simulink model "IEEE9Buses"  (R2024b)
settings: Solver=FixedStepAuto  StartTime=0  StopTime=5  FixedStep=1e-6  RelTol=1e-3
values from neighbouring files (symbols this model uses):
  SG_D_1_D = 0.01056    [SG9_parameters.m]
  SG_D_1_EnableSaturation = 0    [SG9_parameters.m]
  SG_D_1_f0 = 60    [SG9_parameters.m]
  SG_D_1_H = 7.5    [SG9_parameters.m]
  SG_D_1_K_A = 20    [SG9_parameters.m]
  SG_D_1_K_E = 1.000000e+1    (= 10)    [SG9_parameters.m]
  SG_D_1_K_F = 2.363    [SG9_parameters.m]
  SG_D_1_K_s = 5    [SG9_parameters.m]
  SG_D_1_R_a = 0.001088    [SG9_parameters.m]
  SG_D_1_S_A = 1    [SG9_parameters.m]
  SG_D_1_S_B = 0.103    [SG9_parameters.m]
  SG_D_1_S_N = 10.659857    [SG9_parameters.m]
  SG_D_1_SpeedPara = 200    [SG9_parameters.m]
  SG_D_1_T_0 = 0.720173    [SG9_parameters.m]
  SG_D_1_T_1 = 0.3    [SG9_parameters.m]
  SG_D_1_T_2 = 0.05    [SG9_parameters.m]
  SG_D_1_T_3 = 0.02    [SG9_parameters.m]
  SG_D_1_T_4 = 0.005    [SG9_parameters.m]
  SG_D_1_T_A = 0.02    [SG9_parameters.m]
  SG_D_1_T_dd = 8.000000e+0    (= 8)    [SG9_parameters.m]
  SG_D_1_T_ddd = 0.04    [SG9_parameters.m]
  SG_D_1_T_E = 0.314    [SG9_parameters.m]
  SG_D_1_T_F = 0.35    [SG9_parameters.m]
  SG_D_1_T_qd = 0.8    [SG9_parameters.m]
  SG_D_1_T_qdd = 0.02    [SG9_parameters.m]
  SG_D_1_T_speed = 0.1    [SG9_parameters.m]
  SG_D_1_T_w = 0.5    [SG9_parameters.m]
  SG_D_1_V_ref = 1.990276    [SG9_parameters.m]
  SG_D_1_w_ref = 376.991118    [SG9_parameters.m]
  SG_D_1_x_d = 1.9    [SG9_parameters.m]
  SG_D_1_x_dd = 0.302    [SG9_parameters.m]
  SG_D_1_x_ddd = 0.204    [SG9_parameters.m]
  SG_D_1_x_l = 0.05    [SG9_parameters.m]
  SG_D_1_x_q = 1.3    [SG9_parameters.m]
  SG_D_1_x_qd = 0.5    [SG9_parameters.m]
  SG_D_1_x_qdd = 0.3    [SG9_parameters.m]
  SG_D_2_D = 0.01056    [SG9_parameters.m]
  SG_D_2_EnableSaturation = 0    [SG9_parameters.m]
  SG_D_2_f0 = 60    [SG9_parameters.m]
  SG_D_2_H = 7.5    [SG9_parameters.m]
  SG_D_2_K_A = 20    [SG9_parameters.m]
  SG_D_2_K_E = 1.000000e+1    (= 10)    [SG9_parameters.m]
  SG_D_2_K_F = 2.363    [SG9_parameters.m]
  SG_D_2_K_s = 0.5    [SG9_parameters.m]
  SG_D_2_R_a = 0.001088    [SG9_parameters.m]
  SG_D_2_S_A = 1    [SG9_parameters.m]
  SG_D_2_S_B = 0.103    [SG9_parameters.m]
  SG_D_2_S_N = 10.659857    [SG9_parameters.m]
  SG_D_2_SpeedPara = 200    [SG9_parameters.m]
  SG_D_2_T_0 = 1.632913    [SG9_parameters.m]
  SG_D_2_T_1 = 0.2    [SG9_parameters.m]
  SG_D_2_T_2 = 0.05    [SG9_parameters.m]
  SG_D_2_T_3 = 0.02    [SG9_parameters.m]
  SG_D_2_T_4 = 0.005    [SG9_parameters.m]
  SG_D_2_T_A = 0.02    [SG9_parameters.m]
  SG_D_2_T_dd = 8.000000e+0    (= 8)    [SG9_parameters.m]
  SG_D_2_T_ddd = 0.04    [SG9_parameters.m]
  SG_D_2_T_E = 0.314    [SG9_parameters.m]
  SG_D_2_T_F = 0.35    [SG9_parameters.m]
  SG_D_2_T_qd = 0.8    [SG9_parameters.m]
  SG_D_2_T_qdd = 0.02    [SG9_parameters.m]
  SG_D_2_T_speed = 0.1    [SG9_parameters.m]
  SG_D_2_T_w = 0.5    [SG9_parameters.m]
  SG_D_2_V_ref = 2.662631    [SG9_parameters.m]
  SG_D_2_w_ref = 376.991118    [SG9_parameters.m]
  SG_D_2_x_d = 1.9    [SG9_parameters.m]
  SG_D_2_x_dd = 0.302    [SG9_parameters.m]
  SG_D_2_x_ddd = 0.204    [SG9_parameters.m]
  SG_D_2_x_l = 0.05    [SG9_parameters.m]
  SG_D_2_x_q = 1.3    [SG9_parameters.m]
  SG_D_2_x_qd = 0.5    [SG9_parameters.m]
  SG_D_2_x_qdd = 0.3    [SG9_parameters.m]
  SG_D_3_D = 0.01056    [SG9_parameters.m]
  SG_D_3_EnableSaturation = 0    [SG9_parameters.m]
  SG_D_3_f0 = 60    [SG9_parameters.m]
  SG_D_3_H = 7.5    [SG9_parameters.m]
  SG_D_3_K_A = 20    [SG9_parameters.m]
  SG_D_3_K_E = 1.000000e+1    (= 10)    [SG9_parameters.m]
  SG_D_3_K_F = 2.363    [SG9_parameters.m]
  SG_D_3_K_s = 0.5    [SG9_parameters.m]
  SG_D_3_R_a = 0.001088    [SG9_parameters.m]
  SG_D_3_S_A = 1    [SG9_parameters.m]
  SG_D_3_S_B = 0.103    [SG9_parameters.m]
  SG_D_3_S_N = 10.659857    [SG9_parameters.m]
  SG_D_3_SpeedPara = 200    [SG9_parameters.m]
  SG_D_3_T_0 = 0.850788    [SG9_parameters.m]
  SG_D_3_T_1 = 0.2    [SG9_parameters.m]
  SG_D_3_T_2 = 0.05    [SG9_parameters.m]
  SG_D_3_T_3 = 0.02    [SG9_parameters.m]
  SG_D_3_T_4 = 0.005    [SG9_parameters.m]
  SG_D_3_T_A = 0.02    [SG9_parameters.m]
  SG_D_3_T_dd = 8.000000e+0    (= 8)    [SG9_parameters.m]
  SG_D_3_T_ddd = 0.04    [SG9_parameters.m]
  SG_D_3_T_E = 0.314    [SG9_parameters.m]
  SG_D_3_T_F = 0.35    [SG9_parameters.m]
  SG_D_3_T_qd = 0.8    [SG9_parameters.m]
  SG_D_3_T_qdd = 0.02    [SG9_parameters.m]
  SG_D_3_T_speed = 0.1    [SG9_parameters.m]
  SG_D_3_T_w = 0.5    [SG9_parameters.m]
  SG_D_3_V_ref = 1.915682    [SG9_parameters.m]
  SG_D_3_w_ref = 376.991118    [SG9_parameters.m]
  SG_D_3_x_d = 1.9    [SG9_parameters.m]
  SG_D_3_x_dd = 0.302    [SG9_parameters.m]
  SG_D_3_x_ddd = 0.204    [SG9_parameters.m]
  SG_D_3_x_l = 0.05    [SG9_parameters.m]
  SG_D_3_x_q = 1.3    [SG9_parameters.m]
  SG_D_3_x_qd = 0.5    [SG9_parameters.m]
  SG_D_3_x_qdd = 0.3    [SG9_parameters.m]
(part 6 of 9)

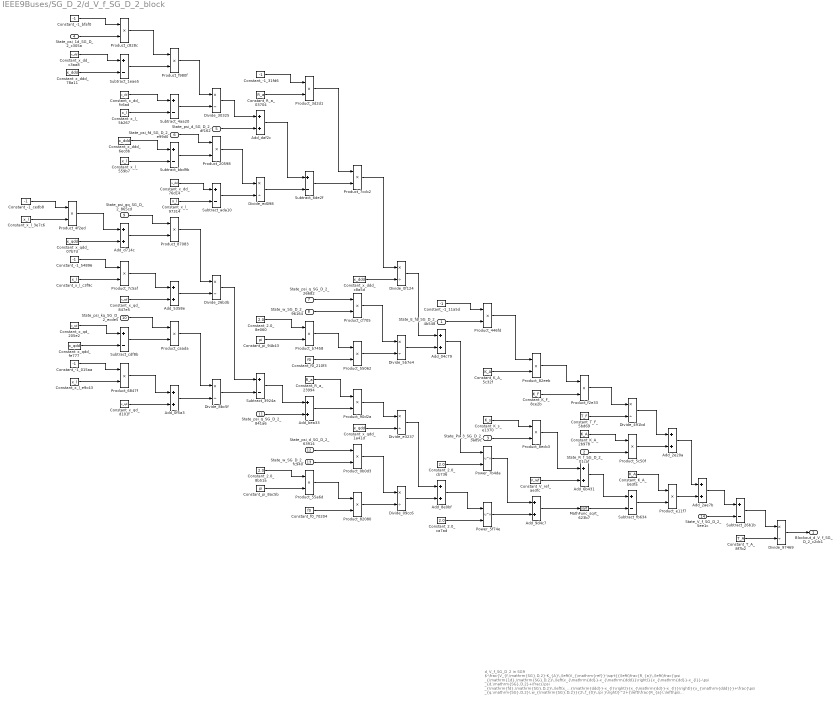
== system IEEE9Buses/SG_D_2/d_V_f_SG_D_2_block ==
  note: d_V_f_SG_D_2 in SG9
      | $-\frac{V_{f,\mathrm{SG},D,2}-K_{A}\,\left(V_{\mathrm{ref}}-\sqrt{{\left(\frac{R_{a}\,\left(\frac{\psi _{\mathrm{1d},\mathrm{SG},D,2}\,\left(x_{\mathrm{dd}}-x_{\mathrm{ddd}}\right)}{x_{\mathrm{dd}}-x_{l}}-\psi _{d,\mathrm{SG},D,2}+\frac{\psi _{\mathrm{fd},\mathrm{SG},D,2}\,\left(x_{\mathrm{ddd}}-x_{l}\right)}{x_{\mathrm{dd}}-x_{l}}\right)}{x_{\mathrm{ddd}}}+\frac{\psi _{q,\mathrm{SG},D,2}\,w_{\mathrm{SG},D,2}}{2\,f_{0}\,\pi }\right)}^2+{\left(\frac{R_{a}\,\left(\psi _{q,\mathrm{SG},D,2}+\frac{\psi _{\mathrm{gq},\mathrm{SG},D,2}\,\left(x_{l}-x_{\mathrm{qdd}}\right)}{x_{l}-x_{\mathrm{qd}}}+\frac{\psi _{\mathrm{kq},\mathrm{SG},D,2}\,\left(x_{\mathrm{qd}}-x_{\mathrm{qdd}}\right)}{x_{l}-x_{\mathrm{qd}}}\right)}{x_{\mathrm{qdd}}}+\frac{\psi _{d,\mathrm{SG},D,2}\,w_{\mathrm{SG},D,2}}{2\,f_{0}\,\pi }\right)}^2}+K_{s}\,\mathrm{Px}_{3,\mathrm{SG},D,2}\right)-K_{A}\,R_{f,\mathrm{SG},D,2}+\frac{E_{\mathrm{fd},\mathrm{SG},D,2}\,K_{A}\,K_{F}}{T_{F}}}{T_{A}}$
      | Automatically generated on 2025-09-12 21:32:35 .
  State_E_fd_SG_D_2_4b548 : Inport
  State_R_f_SG_D_2_01caf : Inport  Port=2
  State_Px_3_SG_D_2_3a89c : Inport  Port=3
  State_psi_1d_SG_D_2_c305a : Inport  Port=4
  State_psi_d_SG_D_2_df162 : Inport  Port=5
  State_psi_fd_SG_D_2_e99d0 : Inport  Port=6
  State_psi_q_SG_D_2_26682 : Inport  Port=7
  State_w_SG_D_2_96164 : Inport  Port=8
  State_psi_gq_SG_D_2_865cd : Inport  Port=9
  State_psi_kq_SG_D_2_ecde5 : Inport  Port=10
  State_psi_q_SG_D_2_841a6 : Inport  Port=11
  State_psi_d_SG_D_2_63914 : Inport  Port=12
  State_w_SG_D_2_fc940 : Inport  Port=13
  State_V_f_SG_D_2_5ee1c : Inport  Port=14
  Add_04c79 : Sum
  Add_0f5a3 : Sum
  Add_2ae7b : Sum
  Add_2e20a : Sum
  Add_5358e : Sum
  Add_6b431 : Sum
  Add_8e0bf : Sum
  Add_9d4c7 : Sum
  Add_bea33 : Sum
  Add_d714c : Sum
  Add_daf2c : Sum
  Constant_-1_015aa : Constant  Value=-1
  Constant_-1_11a5d : Constant  Value=-1
  Constant_-1_31fd6 : Constant  Value=-1
  Constant_-1_54896 : Constant  Value=-1
  Constant_-1_bfaf0 : Constant  Value=-1
  Constant_-1_cedb8 : Constant  Value=-1
  Constant_2.0_8b51a : Constant  Value=2.0
  Constant_2.0_8e060 : Constant  Value=2.0
  Constant_2.0_ca7ad : Constant  Value=2.0
  Constant_2.0_cb736 : Constant  Value=2.0
  Constant_K_A_2b978 : Constant  Value=K_A
  Constant_K_A_5c32f : Constant  Value=K_A
  Constant_K_A_b63fa : Constant  Value=K_A
  Constant_K_F_8ce2b : Constant  Value=K_F
  Constant_K_s_e1370 : Constant  Value=K_s
  Constant_R_a_03704 : Constant  Value=R_a
  Constant_R_a_23994 : Constant  Value=R_a
  Constant_T_A_8f7b2 : Constant  Value=T_A
  Constant_T_F_5bd69 : Constant  Value=T_F
  Constant_V_ref_ae3fc : Constant  Value=V_ref
  Constant_f0_210f3 : Constant  Value=f0
  Constant_f0_70204 : Constant  Value=f0
  Constant_pi_8ac5b : Constant  Value=pi
  Constant_pi_94b43 : Constant  Value=pi
  Constant_x_dd_76d14 : Constant  Value=x_dd
  Constant_x_dd_c3aa8 : Constant  Value=x_dd
  Constant_x_dd_fc6ad : Constant  Value=x_dd
  Constant_x_ddd_6ec8b : Constant  Value=x_ddd
  Constant_x_ddd_78a11 : Constant  Value=x_ddd
  Constant_x_ddd_c8a5d : Constant  Value=x_ddd
  Constant_x_l_3e7c6 : Constant  Value=x_l
  Constant_x_l_559b7 : Constant  Value=x_l
  Constant_x_l_5b267 : Constant  Value=x_l
  Constant_x_l_97314 : Constant  Value=x_l
  Constant_x_l_c3f9c : Constant  Value=x_l
  Constant_x_l_e9c43 : Constant  Value=x_l
  Constant_x_qd_205e2 : Constant  Value=x_qd
  Constant_x_qd_847e5 : Constant  Value=x_qd
  Constant_x_qd_d101f : Constant  Value=x_qd
  Constant_x_qdd_07b7d : Constant  Value=x_qdd
  Constant_x_qdd_1a41d : Constant  Value=x_qdd
  Constant_x_qdd_fe777 : Constant  Value=x_qdd
  Divide_09cc6 : Product  Inputs=*/
  Divide_0f124 : Product  Inputs=*/
  Divide_26b3b : Product  Inputs=*/
  Divide_30325 : Product  Inputs=*/
  Divide_491bd : Product  Inputs=*/
  Divide_5b7e4 : Product  Inputs=*/
  Divide_8bc5f : Product  Inputs=*/
  Divide_97469 : Product  Inputs=*/
  Divide_e3237 : Product  Inputs=*/
  Divide_ed098 : Product  Inputs=*/
  MathFunc_sqrt_623b7 : Sqrt
  Power_5f74e : Math  Operator=pow
  Power_7b4da : Math  Operator=pow
  Product_0b0d3 : Product
  Product_{20598,55062,82080,87083} (4 alike) : Product
  Product_3d2d1 : Product
  Product_446fd : Product
  Product_4f2ed : Product
  Product_55a6d : Product
  Product_5c50f : Product
  Product_6847f : Product
  Product_7c5af : Product
  Product_7ccb2 : Product
  Product_82eeb : Product
  Product_8ecb3 : Product
  Product_90d2a : Product
  Product_b7458 : Product
  Product_c828c : Product
  Product_caada : Product
  Product_cf705 : Product
  Product_e11f7 : Product
  Product_f2e33 : Product
  Product_f980f : Product
  Subtract_1eae5 : Sum  Inputs=+-
  Subtract_26b1b : Sum  Inputs=+-
  Subtract_3924a : Sum  Inputs=+-
  Subtract_4aa20 : Sum  Inputs=+-
  Subtract_6de2f : Sum  Inputs=+-
  Subtract_ada10 : Sum  Inputs=+-
  Subtract_bbd9b : Sum  Inputs=+-
  Subtract_cdf8b : Sum  Inputs=+-
  Subtract_fb634 : Sum  Inputs=+-
  Blockout_d_V_f_SG_D_2_c2dc1 : Outport
  wires:
  Constant_-1_bfaf0/1 -> Product_c828c/1
  Constant_2.0_8e060/1 -> Product_b7458/1
  Constant_-1_cedb8/1 -> Product_4f2ed/1
  Product_b7458/1 -> Product_55062/1
  Product_4f2ed/1 -> Add_d714c/1
  Constant_x_l_e9c43/1 -> Product_6847f/2
  Constant_x_l_3e7c6/1 -> Product_4f2ed/2
  State_psi_1d_SG_D_2_c305a/1 -> Product_c828c/2
  Constant_x_l_97314/1 -> Subtract_ada10/2
  Constant_x_dd_c3aa8/1 -> Subtract_1eae5/1
  Product_90d2a/1 -> Divide_e3237/1
  Constant_x_ddd_78a11/1 -> Subtract_1eae5/2
  Constant_x_qd_d101f/1 -> Add_0f5a3/2
  Add_d714c/1 -> Product_87083/2
  Constant_x_qdd_07b7d/1 -> Add_d714c/2
  Constant_-1_54896/1 -> Product_7c5af/1
  Constant_x_dd_76d14/1 -> Subtract_ada10/1
  Subtract_3924a/1 -> Add_bea33/1
  Power_7b4da/1 -> Add_9d4c7/1
  Constant_x_l_c3f9c/1 -> Product_7c5af/2
  Constant_2.0_8b51a/1 -> Product_55a6d/1
  Constant_x_qd_205e2/1 -> Subtract_cdf8b/1
  Constant_pi_8ac5b/1 -> Product_55a6d/2
  Subtract_6de2f/1 -> Product_7ccb2/2
  Constant_x_qdd_fe777/1 -> Subtract_cdf8b/2
  State_psi_fd_SG_D_2_e99d0/1 -> Product_20598/1
  Constant_-1_015aa/1 -> Product_6847f/1
  Product_c828c/1 -> Product_f980f/1
  State_w_SG_D_2_fc940/1 -> Product_0b0d3/2
  Subtract_1eae5/1 -> Product_f980f/2
  Constant_x_dd_fc6ad/1 -> Subtract_4aa20/1
  State_psi_q_SG_D_2_841a6/1 -> Add_bea33/2
  State_w_SG_D_2_96164/1 -> Product_cf705/2
  Subtract_bbd9b/1 -> Product_20598/2
  Constant_x_l_5b267/1 -> Subtract_4aa20/2
  Add_2e20a/1 -> Add_2ae7b/1
  Constant_x_ddd_6ec8b/1 -> Subtract_bbd9b/1
  Constant_x_l_559b7/1 -> Subtract_bbd9b/2
  State_psi_gq_SG_D_2_865cd/1 -> Product_87083/1
  Product_7c5af/1 -> Add_5358e/1
  Subtract_ada10/1 -> Divide_ed098/2
  Constant_x_qd_847e5/1 -> Add_5358e/2
  Product_cf705/1 -> Divide_5b7e4/1
  State_psi_kq_SG_D_2_ecde5/1 -> Product_caada/1
  Subtract_cdf8b/1 -> Product_caada/2
  Product_20598/1 -> Divide_ed098/1
  State_V_f_SG_D_2_5ee1c/1 -> Subtract_26b1b/2
  Product_6847f/1 -> Add_0f5a3/1
  Product_f980f/1 -> Divide_30325/1
  Divide_26b3b/1 -> Subtract_3924a/1
  Subtract_4aa20/1 -> Divide_30325/2
  Product_87083/1 -> Divide_26b3b/1
  Add_5358e/1 -> Divide_26b3b/2
  Product_caada/1 -> Divide_8bc5f/1
  Divide_ed098/1 -> Subtract_6de2f/2
  Constant_f0_210f3/1 -> Product_55062/2
  Add_0f5a3/1 -> Divide_8bc5f/2
  Divide_30325/1 -> Add_daf2c/1
  State_psi_d_SG_D_2_df162/1 -> Add_daf2c/2
  Divide_8bc5f/1 -> Subtract_3924a/2
  Constant_-1_31fd6/1 -> Product_3d2d1/1
  Constant_R_a_03704/1 -> Product_3d2d1/2
  Constant_f0_70204/1 -> Product_82080/2
  Add_daf2c/1 -> Subtract_6de2f/1
  Product_3d2d1/1 -> Product_7ccb2/1
  Constant_pi_94b43/1 -> Product_b7458/2
  State_psi_q_SG_D_2_26682/1 -> Product_cf705/1
  Constant_R_a_23994/1 -> Product_90d2a/1
  State_E_fd_SG_D_2_4b548/1 -> Product_446fd/2
  Add_bea33/1 -> Product_90d2a/2
  State_psi_d_SG_D_2_63914/1 -> Product_0b0d3/1
  Product_55a6d/1 -> Product_82080/1
  Product_7ccb2/1 -> Divide_0f124/1
  Constant_x_ddd_c8a5d/1 -> Divide_0f124/2
  Product_55062/1 -> Divide_5b7e4/2
  Constant_x_qdd_1a41d/1 -> Divide_e3237/2
  Product_0b0d3/1 -> Divide_09cc6/1
  Product_82080/1 -> Divide_09cc6/2
  Divide_0f124/1 -> Add_04c79/1
  Divide_5b7e4/1 -> Add_04c79/2
  Divide_e3237/1 -> Add_8e0bf/1
  Divide_09cc6/1 -> Add_8e0bf/2
  Constant_-1_11a5d/1 -> Product_446fd/1
  Add_04c79/1 -> Power_7b4da/1
  Constant_2.0_cb736/1 -> Power_7b4da/2
  Add_8e0bf/1 -> Power_5f74e/1
  Constant_2.0_ca7ad/1 -> Power_5f74e/2
  Product_446fd/1 -> Product_82eeb/1
  Constant_K_A_5c32f/1 -> Product_82eeb/2
  Constant_K_s_e1370/1 -> Product_8ecb3/1
  State_Px_3_SG_D_2_3a89c/1 -> Product_8ecb3/2
  Power_5f74e/1 -> Add_9d4c7/2
  Product_82eeb/1 -> Product_f2e33/1
  Constant_K_F_8ce2b/1 -> Product_f2e33/2
  Product_8ecb3/1 -> Add_6b431/1
  Constant_V_ref_ae3fc/1 -> Add_6b431/2
  Add_9d4c7/1 -> MathFunc_sqrt_623b7/1
  Product_f2e33/1 -> Divide_491bd/1
  Constant_T_F_5bd69/1 -> Divide_491bd/2
  Constant_K_A_2b978/1 -> Product_5c50f/1
  State_R_f_SG_D_2_01caf/1 -> Product_5c50f/2
  Add_6b431/1 -> Subtract_fb634/1
  MathFunc_sqrt_623b7/1 -> Subtract_fb634/2
  Divide_491bd/1 -> Add_2e20a/1
  Product_5c50f/1 -> Add_2e20a/2
  Constant_K_A_b63fa/1 -> Product_e11f7/1
  Subtract_fb634/1 -> Product_e11f7/2
  Product_e11f7/1 -> Add_2ae7b/2
  Add_2ae7b/1 -> Subtract_26b1b/1
  Subtract_26b1b/1 -> Divide_97469/1
  Constant_T_A_8f7b2/1 -> Divide_97469/2
  Divide_97469/1 -> Blockout_d_V_f_SG_D_2_c2dc1/1

== system IEEE9Buses/SG_D_2/d_psi_1d_SG_D_2_block ==
  note: d_psi_1d_SG_D_2 in SG9
      | $-\frac{\psi _{\mathrm{1d},\mathrm{SG},D,2}-\psi _{\mathrm{fd},\mathrm{SG},D,2}+\frac{\left(x_{\mathrm{dd}}-x_{l}\right)\,\left(\frac{\psi _{\mathrm{1d},\mathrm{SG},D,2}\,\left(x_{\mathrm{dd}}-x_{\mathrm{ddd}}\right)}{x_{\mathrm{dd}}-x_{l}}-\psi _{d,\mathrm{SG},D,2}+\frac{\psi _{\mathrm{fd},\mathrm{SG},D,2}\,\left(x_{\mathrm{ddd}}-x_{l}\right)}{x_{\mathrm{dd}}-x_{l}}\right)}{x_{\mathrm{ddd}}}}{T_{\mathrm{ddd}}}$
      | Automatically generated on 2025-09-12 21:32:11 .
  State_psi_1d_SG_D_2_680ce : Inport
  State_psi_fd_SG_D_2_d51f2 : Inport  Port=2
  State_psi_1d_SG_D_2_eff8f : Inport  Port=3
  State_psi_d_SG_D_2_8d92a : Inport  Port=4
  State_psi_fd_SG_D_2_13ea5 : Inport  Port=5
  Add_03a29 : Sum
  Add_b8186 : Sum
  Add_c1586 : Sum
  Constant_-1_0798c : Constant  Value=-1
  Constant_-1_a1c61 : Constant  Value=-1
  Constant_T_ddd_58b02 : Constant  Value=T_ddd
  Constant_x_dd_38018 : Constant  Value=x_dd
  Constant_x_dd_39455 : Constant  Value=x_dd
  Constant_x_dd_60610 : Constant  Value=x_dd
  Constant_x_dd_f18ee : Constant  Value=x_dd
  Constant_x_ddd_96c79 : Constant  Value=x_ddd
  Constant_x_ddd_acac6 : Constant  Value=x_ddd
  Constant_x_ddd_b3f94 : Constant  Value=x_ddd
  Constant_x_l_9ac94 : Constant  Value=x_l
  Constant_x_l_a4204 : Constant  Value=x_l
  Constant_x_l_b068a : Constant  Value=x_l
  Constant_x_l_b88a9 : Constant  Value=x_l
  Divide_632b9 : Product  Inputs=*/
  Divide_63f74 : Product  Inputs=*/
  Divide_a9c56 : Product  Inputs=*/
  Divide_c0c5e : Product  Inputs=*/
  Product_52b7e : Product
  Product_67e22 : Product
  Product_72383 : Product
  Product_9b7f5 : Product
  Product_a1c81 : Product
  Subtract_1b96a : Sum  Inputs=+-
  Subtract_2c004 : Sum  Inputs=+-
  Subtract_2cf56 : Sum  Inputs=+-
  Subtract_4de1f : Sum  Inputs=+-
  Subtract_7fdf0 : Sum  Inputs=+-
  Subtract_d0b1e : Sum  Inputs=+-
  Blockout_d_psi_1d_SG_D_2_990c9 : Outport
  wires:
  Subtract_d0b1e/1 -> Product_a1c81/2
  Constant_x_l_b068a/1 -> Subtract_7fdf0/2
  Divide_c0c5e/1 -> Add_b8186/2
  Subtract_2cf56/1 -> Product_52b7e/2
  Constant_-1_0798c/1 -> Product_67e22/1
  Constant_x_dd_f18ee/1 -> Subtract_2c004/1
  Divide_632b9/1 -> Blockout_d_psi_1d_SG_D_2_990c9/1
  State_psi_fd_SG_D_2_d51f2/1 -> Add_03a29/2
  State_psi_1d_SG_D_2_eff8f/1 -> Product_67e22/2
  Divide_63f74/1 -> Subtract_2cf56/2
  Constant_x_ddd_acac6/1 -> Subtract_2c004/2
  State_psi_1d_SG_D_2_680ce/1 -> Product_9b7f5/2
  Product_67e22/1 -> Product_72383/1
  Subtract_2c004/1 -> Product_72383/2
  Constant_x_dd_38018/1 -> Subtract_7fdf0/1
  Constant_x_ddd_96c79/1 -> Subtract_d0b1e/1
  Constant_x_l_a4204/1 -> Subtract_d0b1e/2
  Product_72383/1 -> Divide_a9c56/1
  Subtract_7fdf0/1 -> Divide_a9c56/2
  State_psi_fd_SG_D_2_13ea5/1 -> Product_a1c81/1
  Constant_x_dd_60610/1 -> Subtract_1b96a/1
  Constant_x_l_b88a9/1 -> Subtract_4de1f/2
  Constant_x_l_9ac94/1 -> Subtract_1b96a/2
  Constant_x_ddd_b3f94/1 -> Divide_c0c5e/2
  Divide_a9c56/1 -> Add_c1586/1
  State_psi_d_SG_D_2_8d92a/1 -> Add_c1586/2
  Product_a1c81/1 -> Divide_63f74/1
  Subtract_1b96a/1 -> Divide_63f74/2
  Constant_x_dd_39455/1 -> Subtract_4de1f/1
  Add_c1586/1 -> Subtract_2cf56/1
  Constant_-1_a1c61/1 -> Product_9b7f5/1
  Subtract_4de1f/1 -> Product_52b7e/1
  Product_9b7f5/1 -> Add_03a29/1
  Product_52b7e/1 -> Divide_c0c5e/1
  Add_03a29/1 -> Add_b8186/1
  Add_b8186/1 -> Divide_632b9/1
  Constant_T_ddd_58b02/1 -> Divide_632b9/2

== system IEEE9Buses/SG_D_2/d_psi_d_SG_D_2_block ==
  note: d_psi_d_SG_D_2 in SG9
      | $2\,\pi \,f_{0}\,\left(v_{d,\mathrm{SG},D,2}\,\sin\left(\theta _{\mathrm{SG},D,2}\right)-v_{q,\mathrm{SG},D,2}\,\cos\left(\theta _{\mathrm{SG},D,2}\right)+\frac{R_{a}\,\left(\frac{\psi _{\mathrm{1d},\mathrm{SG},D,2}\,\left(x_{\mathrm{dd}}-x_{\mathrm{ddd}}\right)}{x_{\mathrm{dd}}-x_{l}}-\psi _{d,\mathrm{SG},D,2}+\frac{\psi _{\mathrm{fd},\mathrm{SG},D,2}\,\left(x_{\mathrm{ddd}}-x_{l}\right)}{x_{\mathrm{dd}}-x_{l}}\right)}{x_{\mathrm{ddd}}}+\frac{\psi _{q,\mathrm{SG},D,2}\,w_{\mathrm{SG},D,2}}{2\,f_{0}\,\pi }\right)$
      | Automatically generated on 2025-09-12 21:32:00 .
  State_psi_1d_SG_D_2_5b4b1 : Inport
  State_psi_d_SG_D_2_c6699 : Inport  Port=2
  State_psi_fd_SG_D_2_fabe7 : Inport  Port=3
  Input_v_d_SG_D_2_823c1 : Inport  Port=4
  State_theta_SG_D_2_159ac : Inport  Port=5
  Input_v_q_SG_D_2_1fb2d : Inport  Port=6
  State_theta_SG_D_2_af1f0 : Inport  Port=7
  State_psi_q_SG_D_2_0c26a : Inport  Port=8
  State_w_SG_D_2_33168 : Inport  Port=9
  Add_719cd : Sum
  Add_f3052 : Sum
  Constant_-1_c5ff6 : Constant  Value=-1
  Constant_-2.0_2afdc : Constant  Value=-2.0
  Constant_2.0_7b90a : Constant  Value=2.0
  Constant_R_a_40d35 : Constant  Value=R_a
  Constant_f0_73803 : Constant  Value=f0
  Constant_f0_f2a10 : Constant  Value=f0
  Constant_pi_561d4 : Constant  Value=pi
  Constant_pi_f428f : Constant  Value=pi
  Constant_x_dd_3e231 : Constant  Value=x_dd
  Constant_x_dd_6c3b6 : Constant  Value=x_dd
  Constant_x_dd_af074 : Constant  Value=x_dd
  Constant_x_ddd_28ecd : Constant  Value=x_ddd
  Constant_x_ddd_7f8be : Constant  Value=x_ddd
  Constant_x_ddd_87ec8 : Constant  Value=x_ddd
  Constant_x_l_124f4 : Constant  Value=x_l
  Constant_x_l_23dc5 : Constant  Value=x_l
  Constant_x_l_321d3 : Constant  Value=x_l
  Divide_24f8c : Product  Inputs=*/
  Divide_6a3c1 : Product  Inputs=*/
  Divide_d428a : Product  Inputs=*/
  Divide_f9633 : Product  Inputs=*/
  MathFunc_cos_28cf6 : Trigonometry  Operator=cos
  MathFunc_sin_e82f8 : Trigonometry
  Product_06f7e : Product
  Product_07605 : Product
  Product_1aa22 : Product
  Product_3aa0c : Product
  Product_45316 : Product
  Product_49636 : Product
  Product_4e0df : Product
  Product_8b40d : Product
  Product_988d2 : Product
  Product_aec28 : Product
  Product_c2fde : Product
  Product_d805f : Product
  Subtract_0ddcf : Sum  Inputs=+-
  Subtract_2a1e7 : Sum  Inputs=+-
  Subtract_2bd1a : Sum  Inputs=+-
  Subtract_471cd : Sum  Inputs=+-
  Subtract_81339 : Sum  Inputs=+-
  Subtract_a4411 : Sum  Inputs=+-
  Subtract_bce5a : Sum  Inputs=+-
  Blockout_d_psi_d_SG_D_2_d579c : Outport
  wires:
  MathFunc_sin_e82f8/1 -> Product_3aa0c/2
  Constant_x_dd_3e231/1 -> Subtract_471cd/1
  Constant_-1_c5ff6/1 -> Product_aec28/1
  Constant_x_l_124f4/1 -> Subtract_471cd/2
  State_psi_1d_SG_D_2_5b4b1/1 -> Product_aec28/2
  Constant_f0_73803/1 -> Product_1aa22/2
  Constant_2.0_7b90a/1 -> Product_c2fde/1
  Constant_x_l_23dc5/1 -> Subtract_81339/2
  Constant_x_dd_6c3b6/1 -> Subtract_0ddcf/1
  Product_07605/1 -> Blockout_d_psi_d_SG_D_2_d579c/1
  Constant_pi_f428f/1 -> Product_c2fde/2
  Constant_x_ddd_87ec8/1 -> Subtract_0ddcf/2
  Subtract_2a1e7/1 -> Product_07605/2
  Product_aec28/1 -> Product_49636/1
  Product_c2fde/1 -> Product_d805f/1
  Subtract_0ddcf/1 -> Product_49636/2
  Divide_f9633/1 -> Subtract_2a1e7/2
  Constant_x_ddd_7f8be/1 -> Subtract_bce5a/1
  Constant_x_l_321d3/1 -> Subtract_bce5a/2
  Product_49636/1 -> Divide_d428a/1
  Subtract_2bd1a/1 -> Add_719cd/1
  Subtract_471cd/1 -> Divide_d428a/2
  State_psi_fd_SG_D_2_fabe7/1 -> Product_45316/1
  Subtract_bce5a/1 -> Product_45316/2
  Constant_x_dd_af074/1 -> Subtract_81339/1
  Divide_d428a/1 -> Add_f3052/1
  State_psi_d_SG_D_2_c6699/1 -> Add_f3052/2
  Product_45316/1 -> Divide_6a3c1/1
  Subtract_81339/1 -> Divide_6a3c1/2
  Add_f3052/1 -> Subtract_a4411/1
  Divide_6a3c1/1 -> Subtract_a4411/2
  Constant_R_a_40d35/1 -> Product_4e0df/1
  Subtract_a4411/1 -> Product_4e0df/2
  Divide_24f8c/1 -> Subtract_2bd1a/1
  State_theta_SG_D_2_159ac/1 -> MathFunc_sin_e82f8/1
  Product_4e0df/1 -> Divide_24f8c/1
  Constant_-2.0_2afdc/1 -> Product_988d2/1
  Input_v_d_SG_D_2_823c1/1 -> Product_3aa0c/1
  Constant_x_ddd_28ecd/1 -> Divide_24f8c/2
  State_theta_SG_D_2_af1f0/1 -> MathFunc_cos_28cf6/1
  Product_1aa22/1 -> Product_07605/1
  Product_3aa0c/1 -> Subtract_2bd1a/2
  Product_988d2/1 -> Product_1aa22/1
  Input_v_q_SG_D_2_1fb2d/1 -> Product_06f7e/1
  MathFunc_cos_28cf6/1 -> Product_06f7e/2
  State_psi_q_SG_D_2_0c26a/1 -> Product_8b40d/1
  State_w_SG_D_2_33168/1 -> Product_8b40d/2
  Constant_f0_f2a10/1 -> Product_d805f/2
  Constant_pi_561d4/1 -> Product_988d2/2
  Product_06f7e/1 -> Add_719cd/2
  Product_8b40d/1 -> Divide_f9633/1
  Product_d805f/1 -> Divide_f9633/2
  Add_719cd/1 -> Subtract_2a1e7/1

== system IEEE9Buses/SG_D_2/d_psi_fd_SG_D_2_block ==
  note: d_psi_fd_SG_D_2 in SG9
      | $-\frac{\psi _{\mathrm{fd},\mathrm{SG},D,2}-E_{\mathrm{fd},\mathrm{SG},D,2}+\left(x_{d}-x_{\mathrm{dd}}\right)\,\left(\frac{\frac{\psi _{\mathrm{1d},\mathrm{SG},D,2}\,\left(x_{\mathrm{dd}}-x_{\mathrm{ddd}}\right)}{x_{\mathrm{dd}}-x_{l}}-\psi _{d,\mathrm{SG},D,2}+\frac{\psi _{\mathrm{fd},\mathrm{SG},D,2}\,\left(x_{\mathrm{ddd}}-x_{l}\right)}{x_{\mathrm{dd}}-x_{l}}}{x_{\mathrm{ddd}}}-\frac{\left(x_{\mathrm{dd}}-x_{\mathrm{ddd}}\right)\,\left(\psi _{\mathrm{1d},\mathrm{SG},D,2}-\psi _{\mathrm{fd},\mathrm{SG},D,2}+\frac{\left(x_{\mathrm{dd}}-x_{l}\right)\,\left(\frac{\psi _{\mathrm{1d},\mathrm{SG},D,2}\,\left(x_{\mathrm{dd}}-x_{\mathrm{ddd}}\right)}{x_{\mathrm{dd}}-x_{l}}-\psi _{d,\mathrm{SG},D,2}+\frac{\psi _{\mathrm{fd},\mathrm{SG},D,2}\,\left(x_{\mathrm{ddd}}-x_{l}\right)}{x_{\mathrm{dd}}-x_{l}}\right)}{x_{\mathrm{ddd}}}\right)}{{\left(x_{\mathrm{dd}}-x_{l}\right)}^2}\right)}{T_{\mathrm{dd}}}$
      | Automatically generated on 2025-09-12 21:32:08 .
  State_E_fd_SG_D_2_4ddbc : Inport
  State_psi_fd_SG_D_2_7c19b : Inport  Port=2
  State_psi_1d_SG_D_2_ddd99 : Inport  Port=3
  State_psi_fd_SG_D_2_ebd42 : Inport  Port=4
  State_psi_1d_SG_D_2_69a8e : Inport  Port=5
  State_psi_d_SG_D_2_a4eb1 : Inport  Port=6
  State_psi_fd_SG_D_2_d7212 : Inport  Port=7
  State_psi_1d_SG_D_2_6526c : Inport  Port=8
  State_psi_d_SG_D_2_1bf37 : Inport  Port=9
  State_psi_fd_SG_D_2_79a88 : Inport  Port=10
  Add_2c969 : Sum
  Add_83df4 : Sum
  Constant_-1_29111 : Constant  Value=-1
  Constant_-1_675e4 : Constant  Value=-1
  Constant_-1_fd813 : Constant  Value=-1
  Constant_2.0_0fd01 : Constant  Value=2.0
  Constant_T_dd_e31a3 : Constant  Value=T_dd
  Constant_x_d_e14ad : Constant  Value=x_d
  Constant_x_dd_08212 : Constant  Value=x_dd
  Constant_x_dd_23c89 : Constant  Value=x_dd
  Constant_x_dd_4561f : Constant  Value=x_dd
  Constant_x_dd_58acc : Constant  Value=x_dd
  Constant_x_dd_6534d : Constant  Value=x_dd
  Constant_x_dd_6ab1d : Constant  Value=x_dd
  Constant_x_dd_80383 : Constant  Value=x_dd
  Constant_x_dd_83849 : Constant  Value=x_dd
  Constant_x_dd_a989d : Constant  Value=x_dd
  Constant_x_dd_c6904 : Constant  Value=x_dd
  Constant_x_ddd_b8f92 : Constant  Value=x_ddd
  Constant_x_ddd_cde6e : Constant  Value=x_ddd
  Constant_x_ddd_d3684 : Constant  Value=x_ddd
  Constant_x_ddd_d5a52 : Constant  Value=x_ddd
  Constant_x_ddd_e64e8 : Constant  Value=x_ddd
  Constant_x_ddd_eb6ce : Constant  Value=x_ddd
  Constant_x_ddd_ee606 : Constant  Value=x_ddd
  Constant_x_l_778cc : Constant  Value=x_l
  Constant_x_l_8bec8 : Constant  Value=x_l
  Constant_x_l_9a2d6 : Constant  Value=x_l
  Constant_x_l_a30fd : Constant  Value=x_l
  Constant_x_l_a639e : Constant  Value=x_l
  Constant_x_l_c34eb : Constant  Value=x_l
  Constant_x_l_dd9ba : Constant  Value=x_l
  Constant_x_l_ed765 : Constant  Value=x_l
  Divide_29374 : Product  Inputs=*/
  Divide_383bf : Product  Inputs=*/
  Divide_3e31d : Product  Inputs=*/
  Divide_cd552 : Product  Inputs=*/
  Divide_d7dc3 : Product  Inputs=*/
  Divide_d89c5 : Product  Inputs=*/
  Divide_d951d : Product  Inputs=*/
  Divide_f635a : Product  Inputs=*/
  Power_a6ec9 : Math  Operator=pow
  Product_0c75d : Product
  Product_2cefd : Product
  Product_35bdc : Product
  Product_64081 : Product
  Product_65868 : Product
  Product_80095 : Product
  Product_869a6 : Product
  Product_90b2b : Product
  Product_ab7fc : Product
  Product_e1ce9 : Product
  Subtract_10a1e : Sum  Inputs=+-
  Subtract_33c34 : Sum  Inputs=+-
  Subtract_3554d : Sum  Inputs=+-
  Subtract_43f92 : Sum  Inputs=+-
  Subtract_46095 : Sum  Inputs=+-
  Subtract_5d59d : Sum  Inputs=+-
  Subtract_7a495 : Sum  Inputs=+-
  Subtract_92895 : Sum  Inputs=+-
  Subtract_97551 : Sum  Inputs=+-
  Subtract_a3637 : Sum  Inputs=+-
  Subtract_b0fcb : Sum  Inputs=+-
  Subtract_c630a : Sum  Inputs=+-
  Subtract_d4ee7 : Sum  Inputs=+-
  Subtract_d7ab7 : Sum  Inputs=+-
  Subtract_dc16e : Sum  Inputs=+-
  Subtract_dcdb4 : Sum  Inputs=+-
  Subtract_e2a4b : Sum  Inputs=+-
  Subtract_eb7d4 : Sum  Inputs=+-
  Subtract_f0216 : Sum  Inputs=+-
  Blockout_d_psi_fd_SG_D_2_e3965 : Outport
  wires:
  Constant_x_dd_6534d/1 -> Subtract_3554d/1
  Constant_-1_675e4/1 -> Product_ab7fc/1
  Constant_x_l_ed765/1 -> Subtract_7a495/2
  Divide_3e31d/1 -> Add_2c969/1
  Subtract_97551/1 -> Product_80095/2
  Constant_x_l_9a2d6/1 -> Subtract_3554d/2
  Product_80095/1 -> Divide_d89c5/1
  State_psi_1d_SG_D_2_69a8e/1 -> Product_ab7fc/2
  Constant_x_dd_08212/1 -> Subtract_c630a/1
  Product_e1ce9/1 -> Divide_3e31d/1
  Constant_x_dd_c6904/1 -> Subtract_46095/1
  Constant_x_ddd_ee606/1 -> Subtract_c630a/2
  Constant_x_dd_23c89/1 -> Subtract_f0216/1
  Product_ab7fc/1 -> Product_2cefd/1
  Subtract_c630a/1 -> Product_2cefd/2
  State_psi_d_SG_D_2_1bf37/1 -> Add_2c969/2
  Constant_x_ddd_d3684/1 -> Subtract_97551/1
  Constant_x_l_8bec8/1 -> Subtract_97551/2
  Product_2cefd/1 -> Divide_f635a/1
  Subtract_3554d/1 -> Divide_f635a/2
  State_psi_fd_SG_D_2_d7212/1 -> Product_80095/1
  Subtract_d7ab7/1 -> Product_0c75d/2
  Constant_x_dd_6ab1d/1 -> Subtract_d4ee7/1
  Constant_x_l_dd9ba/1 -> Subtract_d4ee7/2
  Product_869a6/1 -> Product_0c75d/1
  Divide_f635a/1 -> Add_83df4/1
  State_psi_d_SG_D_2_a4eb1/1 -> Add_83df4/2
  Subtract_d4ee7/1 -> Divide_d89c5/2
  Constant_x_dd_83849/1 -> Subtract_7a495/1
  Constant_x_ddd_d5a52/1 -> Subtract_eb7d4/1
  Add_83df4/1 -> Subtract_92895/1
  Divide_d89c5/1 -> Subtract_92895/2
  Constant_-1_fd813/1 -> Product_65868/1
  Product_64081/1 -> Divide_383bf/1
  State_psi_1d_SG_D_2_6526c/1 -> Product_65868/2
  Subtract_46095/1 -> Product_869a6/2
  Constant_x_dd_58acc/1 -> Subtract_dcdb4/1
  Divide_383bf/1 -> Subtract_dc16e/2
  Constant_-1_29111/1 -> Product_869a6/1
  Constant_x_ddd_eb6ce/1 -> Subtract_dcdb4/2
  Constant_x_ddd_cde6e/1 -> Divide_d951d/2
  Subtract_7a495/1 -> Product_90b2b/1
  Subtract_92895/1 -> Product_90b2b/2
  State_psi_fd_SG_D_2_ebd42/1 -> Subtract_33c34/2
  Product_65868/1 -> Product_e1ce9/1
  Subtract_dcdb4/1 -> Product_e1ce9/2
  Constant_2.0_0fd01/1 -> Power_a6ec9/2
  State_psi_1d_SG_D_2_ddd99/1 -> Subtract_33c34/1
  Constant_x_dd_4561f/1 -> Subtract_e2a4b/1
  Subtract_eb7d4/1 -> Product_64081/2
  Constant_x_l_c34eb/1 -> Subtract_e2a4b/2
  Constant_x_l_a30fd/1 -> Subtract_eb7d4/2
  Constant_x_ddd_e64e8/1 -> Subtract_46095/2
  Subtract_f0216/1 -> Divide_383bf/2
  Product_90b2b/1 -> Divide_d951d/1
  Subtract_e2a4b/1 -> Divide_3e31d/2
  State_psi_fd_SG_D_2_79a88/1 -> Product_64081/1
  Constant_x_l_a639e/1 -> Subtract_f0216/2
  Constant_x_dd_80383/1 -> Subtract_10a1e/1
  Subtract_33c34/1 -> Subtract_d7ab7/1
  Divide_d951d/1 -> Subtract_d7ab7/2
  Constant_x_l_778cc/1 -> Subtract_10a1e/2
  Subtract_10a1e/1 -> Power_a6ec9/1
  Add_2c969/1 -> Subtract_dc16e/1
  Product_0c75d/1 -> Divide_29374/1
  Power_a6ec9/1 -> Divide_29374/2
  Subtract_dc16e/1 -> Divide_d7dc3/1
  Constant_x_ddd_b8f92/1 -> Divide_d7dc3/2
  Constant_x_d_e14ad/1 -> Subtract_b0fcb/1
  Constant_x_dd_a989d/1 -> Subtract_b0fcb/2
  Divide_29374/1 -> Subtract_a3637/1
  Divide_d7dc3/1 -> Subtract_a3637/2
  State_E_fd_SG_D_2_4ddbc/1 -> Subtract_43f92/1
  State_psi_fd_SG_D_2_7c19b/1 -> Subtract_43f92/2
  Subtract_b0fcb/1 -> Product_35bdc/1
  Subtract_a3637/1 -> Product_35bdc/2
  Subtract_43f92/1 -> Subtract_5d59d/1
  Product_35bdc/1 -> Subtract_5d59d/2
  Subtract_5d59d/1 -> Divide_cd552/1
  Constant_T_dd_e31a3/1 -> Divide_cd552/2
  Divide_cd552/1 -> Blockout_d_psi_fd_SG_D_2_e3965/1

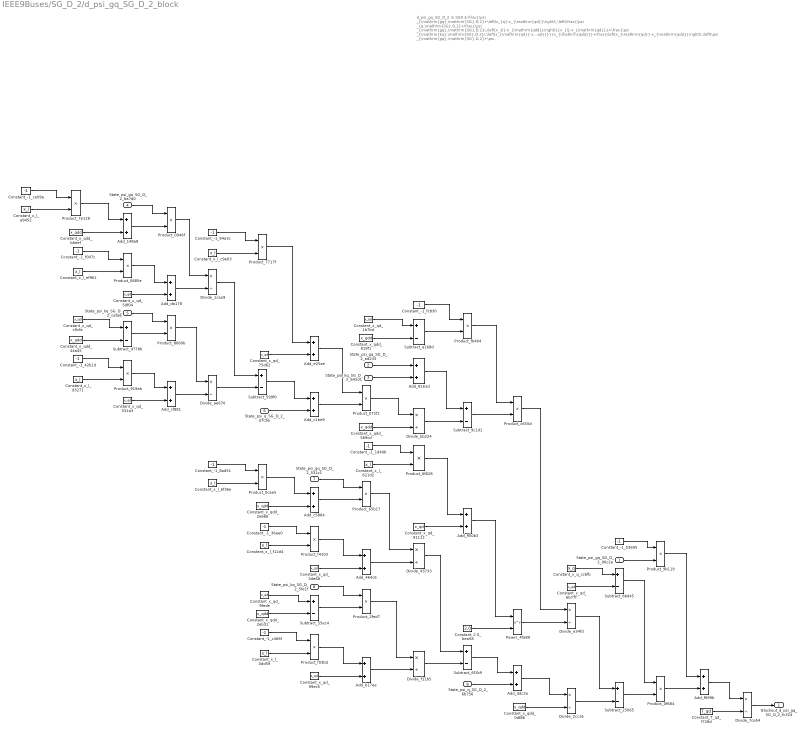
== system IEEE9Buses/SG_D_2/d_psi_gq_SG_D_2_block ==
  note: d_psi_gq_SG_D_2 in SG9
      | $-\frac{\psi _{\mathrm{gq},\mathrm{SG},D,2}+\left(x_{q}-x_{\mathrm{qd}}\right)\,\left(\frac{\psi _{q,\mathrm{SG},D,2}+\frac{\psi _{\mathrm{gq},\mathrm{SG},D,2}\,\left(x_{l}-x_{\mathrm{qdd}}\right)}{x_{l}-x_{\mathrm{qd}}}+\frac{\psi _{\mathrm{kq},\mathrm{SG},D,2}\,\left(x_{\mathrm{qd}}-x_{\mathrm{qdd}}\right)}{x_{l}-x_{\mathrm{qd}}}}{x_{\mathrm{qdd}}}+\frac{\left(x_{\mathrm{qd}}-x_{\mathrm{qdd}}\right)\,\left(\psi _{\mathrm{gq},\mathrm{SG},D,2}+\psi _{\mathrm{kq},\mathrm{SG},D,2}+\frac{\left(x_{l}-x_{\mathrm{qd}}\right)\,\left(\psi _{q,\mathrm{SG},D,2}+\frac{\psi _{\mathrm{gq},\mathrm{SG},D,2}\,\left(x_{l}-x_{\mathrm{qdd}}\right)}{x_{l}-x_{\mathrm{qd}}}+\frac{\psi _{\mathrm{kq},\mathrm{SG},D,2}\,\left(x_{\mathrm{qd}}-x_{\mathrm{qdd}}\right)}{x_{l}-x_{\mathrm{qd}}}\right)}{x_{\mathrm{qdd}}}\right)}{{\left(x_{l}-x_{\mathrm{qd}}\right)}^2}\right)}{T_{\mathrm{qd}}}$
      | Automatically generated on 2025-09-12 21:32:17 .
  State_psi_gq_SG_D_2_06c2a : Inport
  State_psi_gq_SG_D_2_ad233 : Inport  Port=2
  State_psi_kq_SG_D_2_642d1 : Inport  Port=3
  State_psi_gq_SG_D_2_ba7d0 : Inport  Port=4
  State_psi_kq_SG_D_2_cefa6 : Inport  Port=5
  State_psi_q_SG_D_2_d7c9a : Inport  Port=6
  State_psi_gq_SG_D_2_531c1 : Inport  Port=7
  State_psi_kq_SG_D_2_5fe1f : Inport  Port=8
  State_psi_q_SG_D_2_6b756 : Inport  Port=9
  Add_148a8 : Sum
  Add_464c6 : Sum
  Add_8161d : Sum
  Add_950b3 : Sum
  Add_b17ee : Sum
  Add_c1be9 : Sum
  Add_c5864 : Sum
  Add_cf881 : Sum
  Add_da178 : Sum
  Add_ddc2e : Sum
  Add_e25ae : Sum
  Add_f699b : Sum
  Constant_-1_03695 : Constant  Value=-1
  Constant_-1_1d40b : Constant  Value=-1
  Constant_-1_36ae0 : Constant  Value=-1
  Constant_-1_42b1d : Constant  Value=-1
  Constant_-1_8ad51 : Constant  Value=-1
  Constant_-1_94a3c : Constant  Value=-1
  Constant_-1_c466f : Constant  Value=-1
  Constant_-1_ce09a : Constant  Value=-1
  Constant_-1_f007c : Constant  Value=-1
  Constant_-1_fc830 : Constant  Value=-1
  Constant_2.0_bea58 : Constant  Value=2.0
  Constant_T_qd_f728d : Constant  Value=T_qd
  Constant_x_l_0dd59 : Constant  Value=x_l
  Constant_x_l_621d2 : Constant  Value=x_l
  Constant_x_l_6f36e : Constant  Value=x_l
  Constant_x_l_a9452 : Constant  Value=x_l
  Constant_x_l_c9e03 : Constant  Value=x_l
  Constant_x_l_d3271 : Constant  Value=x_l
  Constant_x_l_ef961 : Constant  Value=x_l
  Constant_x_l_f12d4 : Constant  Value=x_l
  Constant_x_q_cc6fb : Constant  Value=x_q
  Constant_x_qd_1b7bd : Constant  Value=x_qd
  Constant_x_qd_3de68 : Constant  Value=x_qd
  Constant_x_qd_531a3 : Constant  Value=x_qd
  Constant_x_qd_5df04 : Constant  Value=x_qd
  Constant_x_qd_6b77f : Constant  Value=x_qd
  Constant_x_qd_75d62 : Constant  Value=x_qd
  Constant_x_qd_91112 : Constant  Value=x_qd
  Constant_x_qd_99ec5 : Constant  Value=x_qd
  Constant_x_qd_9fede : Constant  Value=x_qd
  Constant_x_qd_c9cfa : Constant  Value=x_qd
  Constant_x_qdd_0df86 : Constant  Value=x_qdd
  Constant_x_qdd_2e666 : Constant  Value=x_qdd
  Constant_x_qdd_2eb31 : Constant  Value=x_qdd
  Constant_x_qdd_44a45 : Constant  Value=x_qdd
  Constant_x_qdd_569cd : Constant  Value=x_qdd
  Constant_x_qdd_819f1 : Constant  Value=x_qdd
  Constant_x_qdd_b6eef : Constant  Value=x_qdd
  Divide_1caa9 : Product  Inputs=*/
  Divide_2cc16 : Product  Inputs=*/
  Divide_43733 : Product  Inputs=*/
  Divide_7ce54 : Product  Inputs=*/
  Divide_ae670 : Product  Inputs=*/
  Divide_bb224 : Product  Inputs=*/
  Divide_e34fd : Product  Inputs=*/
  Divide_f11b5 : Product  Inputs=*/
  Power_4fa89 : Math  Operator=pow
  Product_0685e : Product
  Product_072f2 : Product
  Product_0946f : Product
  Product_0cae5 : Product
  Product_0f684 : Product
  Product_2fed7 : Product
  Product_65b17 : Product
  Product_6f628 : Product
  Product_7717f : Product
  Product_7e128 : Product
  Product_8060b : Product
  Product_919ab : Product
  Product_9b119 : Product
  Product_c655d : Product
  Product_f03bd : Product
  Product_f4103 : Product
  Product_fb404 : Product
  Subtract_25065 : Sum  Inputs=+-
  Subtract_55ec4 : Sum  Inputs=+-
  Subtract_599f0 : Sum  Inputs=+-
  Subtract_6bd45 : Sum  Inputs=+-
  Subtract_6f1b9 : Sum  Inputs=+-
  Subtract_9c1d1 : Sum  Inputs=+-
  Subtract_a168d : Sum  Inputs=+-
  Subtract_d778b : Sum  Inputs=+-
  Blockout_d_psi_gq_SG_D_2_fc324 : Outport
  wires:
  Constant_x_l_0dd59/1 -> Product_f03bd/2
  Constant_x_l_6f36e/1 -> Product_0cae5/2
  Constant_x_qd_c9cfa/1 -> Subtract_d778b/1
  Constant_x_l_621d2/1 -> Product_6f628/2
  Constant_x_qdd_819f1/1 -> Subtract_a168d/2
  Constant_-1_42b1d/1 -> Product_919ab/1
  Constant_-1_ce09a/1 -> Product_7e128/1
  State_psi_gq_SG_D_2_ad233/1 -> Add_8161d/1
  Constant_x_qdd_44a45/1 -> Subtract_d778b/2
  Constant_x_qd_1b7bd/1 -> Subtract_a168d/1
  Constant_x_l_d3271/1 -> Product_919ab/2
  Constant_x_l_a9452/1 -> Product_7e128/2
  Product_919ab/1 -> Add_cf881/1
  Product_7e128/1 -> Add_148a8/1
  Constant_x_l_ef961/1 -> Product_0685e/2
  Constant_x_l_c9e03/1 -> Product_7717f/2
  Constant_x_qd_531a3/1 -> Add_cf881/2
  Constant_x_qdd_b6eef/1 -> Add_148a8/2
  Constant_-1_f007c/1 -> Product_0685e/1
  Constant_x_qd_99ec5/1 -> Add_b17ee/2
  Constant_x_qdd_2e666/1 -> Add_c5864/2
  State_psi_gq_SG_D_2_ba7d0/1 -> Product_0946f/1
  Add_cf881/1 -> Divide_ae670/2
  Add_148a8/1 -> Product_0946f/2
  Constant_x_qd_6b77f/1 -> Subtract_6bd45/2
  Product_0685e/1 -> Add_da178/1
  Constant_x_qd_5df04/1 -> Add_da178/2
  State_psi_kq_SG_D_2_cefa6/1 -> Product_8060b/1
  Divide_1caa9/1 -> Subtract_599f0/1
  Subtract_d778b/1 -> Product_8060b/2
  Product_0946f/1 -> Divide_1caa9/1
  Add_da178/1 -> Divide_1caa9/2
  Add_c1be9/1 -> Product_072f2/2
  Product_8060b/1 -> Divide_ae670/1
  Constant_-1_94a3c/1 -> Product_7717f/1
  Divide_ae670/1 -> Subtract_599f0/2
  Constant_-1_c466f/1 -> Product_f03bd/1
  Constant_-1_8ad51/1 -> Product_0cae5/1
  Product_7717f/1 -> Add_e25ae/1
  Constant_x_qdd_2eb31/1 -> Subtract_55ec4/2
  Constant_x_qd_75d62/1 -> Add_e25ae/2
  Subtract_599f0/1 -> Add_c1be9/1
  Constant_-1_1d40b/1 -> Product_6f628/1
  State_psi_q_SG_D_2_d7c9a/1 -> Add_c1be9/2
  Product_f03bd/1 -> Add_b17ee/1
  Product_0cae5/1 -> Add_c5864/1
  Constant_-1_36ae0/1 -> Product_f4103/1
  Product_072f2/1 -> Divide_bb224/1
  Constant_x_l_f12d4/1 -> Product_f4103/2
  Product_0f684/1 -> Add_f699b/2
  Constant_x_qd_9fede/1 -> Subtract_55ec4/1
  Add_e25ae/1 -> Product_072f2/1
  State_psi_gq_SG_D_2_531c1/1 -> Product_65b17/1
  Add_b17ee/1 -> Divide_f11b5/2
  Add_c5864/1 -> Product_65b17/2
  Product_f4103/1 -> Add_464c6/1
  Constant_x_qd_3de68/1 -> Add_464c6/2
  State_psi_kq_SG_D_2_5fe1f/1 -> Product_2fed7/1
  Subtract_55ec4/1 -> Product_2fed7/2
  Divide_f11b5/1 -> Subtract_6f1b9/2
  State_psi_kq_SG_D_2_642d1/1 -> Add_8161d/2
  Product_2fed7/1 -> Divide_f11b5/1
  Constant_x_qdd_569cd/1 -> Divide_bb224/2
  Product_65b17/1 -> Divide_43733/1
  Add_464c6/1 -> Divide_43733/2
  Constant_-1_fc830/1 -> Product_fb404/1
  Subtract_a168d/1 -> Product_fb404/2
  Add_8161d/1 -> Subtract_9c1d1/1
  Divide_bb224/1 -> Subtract_9c1d1/2
  Product_6f628/1 -> Add_950b3/1
  Constant_x_qd_91112/1 -> Add_950b3/2
  Divide_43733/1 -> Subtract_6f1b9/1
  Product_fb404/1 -> Product_c655d/1
  Subtract_9c1d1/1 -> Product_c655d/2
  Add_950b3/1 -> Power_4fa89/1
  Constant_2.0_bea58/1 -> Power_4fa89/2
  Subtract_6f1b9/1 -> Add_ddc2e/1
  State_psi_q_SG_D_2_6b756/1 -> Add_ddc2e/2
  Product_c655d/1 -> Divide_e34fd/1
  Power_4fa89/1 -> Divide_e34fd/2
  Add_ddc2e/1 -> Divide_2cc16/1
  Constant_x_qdd_0df86/1 -> Divide_2cc16/2
  Constant_x_q_cc6fb/1 -> Subtract_6bd45/1
  Divide_e34fd/1 -> Subtract_25065/1
  Divide_2cc16/1 -> Subtract_25065/2
  Divide_7ce54/1 -> Blockout_d_psi_gq_SG_D_2_fc324/1
  Constant_-1_03695/1 -> Product_9b119/1
  State_psi_gq_SG_D_2_06c2a/1 -> Product_9b119/2
  Subtract_6bd45/1 -> Product_0f684/1
  Subtract_25065/1 -> Product_0f684/2
  Product_9b119/1 -> Add_f699b/1
  Add_f699b/1 -> Divide_7ce54/1
  Constant_T_qd_f728d/1 -> Divide_7ce54/2

== system IEEE9Buses/SG_D_2/d_psi_kq_SG_D_2_block ==
  note: d_psi_kq_SG_D_2 in SG9
      | $-\frac{\psi _{\mathrm{gq},\mathrm{SG},D,2}+\psi _{\mathrm{kq},\mathrm{SG},D,2}+\frac{\left(x_{l}-x_{\mathrm{qd}}\right)\,\left(\psi _{q,\mathrm{SG},D,2}+\frac{\psi _{\mathrm{gq},\mathrm{SG},D,2}\,\left(x_{l}-x_{\mathrm{qdd}}\right)}{x_{l}-x_{\mathrm{qd}}}+\frac{\psi _{\mathrm{kq},\mathrm{SG},D,2}\,\left(x_{\mathrm{qd}}-x_{\mathrm{qdd}}\right)}{x_{l}-x_{\mathrm{qd}}}\right)}{x_{\mathrm{qdd}}}}{T_{\mathrm{qdd}}}$
      | Automatically generated on 2025-09-12 21:32:20 .
  State_psi_gq_SG_D_2_2a2b4 : Inport
  State_psi_kq_SG_D_2_3768b : Inport  Port=2
  State_psi_gq_SG_D_2_8a6ac : Inport  Port=3
  State_psi_kq_SG_D_2_dff77 : Inport  Port=4
  State_psi_q_SG_D_2_e662c : Inport  Port=5
  Add_95af3 : Sum
  Add_b0455 : Sum
  Add_baf6a : Sum
  Add_c1458 : Sum
  Add_cf74d : Sum
  Add_da69a : Sum
  Constant_-1_0a86c : Constant  Value=-1
  Constant_-1_2494f : Constant  Value=-1
  Constant_-1_50411 : Constant  Value=-1
  Constant_-1_cf773 : Constant  Value=-1
  Constant_-1_e3414 : Constant  Value=-1
  Constant_T_qdd_05550 : Constant  Value=T_qdd
  Constant_x_l_0c1df : Constant  Value=x_l
  Constant_x_l_3eb2d : Constant  Value=x_l
  Constant_x_l_762a1 : Constant  Value=x_l
  Constant_x_l_b8f3c : Constant  Value=x_l
  Constant_x_qd_683e6 : Constant  Value=x_qd
  Constant_x_qd_98b8a : Constant  Value=x_qd
  Constant_x_qd_cfa97 : Constant  Value=x_qd
  Constant_x_qd_fc460 : Constant  Value=x_qd
  Constant_x_qdd_6591c : Constant  Value=x_qdd
  Constant_x_qdd_c1c90 : Constant  Value=x_qdd
  Constant_x_qdd_cc240 : Constant  Value=x_qdd
  Divide_679ed : Product  Inputs=*/
  Divide_80bed : Product  Inputs=*/
  Divide_84aa8 : Product  Inputs=*/
  Divide_c7b3e : Product  Inputs=*/
  Product_0abff : Product
  Product_2f50c : Product
  Product_35aaa : Product
  Product_b0544 : Product
  Product_b9aec : Product
  Product_dfb4a : Product
  Product_e50dd : Product
  Product_e73d5 : Product
  Subtract_2808a : Sum  Inputs=+-
  Subtract_33998 : Sum  Inputs=+-
  Subtract_94387 : Sum  Inputs=+-
  Blockout_d_psi_kq_SG_D_2_b6d40 : Outport
  wires:
  State_psi_kq_SG_D_2_3768b/1 -> Subtract_94387/2
  Constant_-1_e3414/1 -> Product_e50dd/1
  Constant_-1_0a86c/1 -> Product_b0544/1
  Constant_x_l_762a1/1 -> Product_b0544/2
  Constant_x_qdd_cc240/1 -> Add_b0455/2
  Constant_x_l_0c1df/1 -> Product_e50dd/2
  Constant_x_qd_cfa97/1 -> Subtract_33998/1
  Constant_T_qdd_05550/1 -> Divide_c7b3e/2
  Constant_-1_2494f/1 -> Product_2f50c/1
  Product_b0544/1 -> Add_b0455/1
  Constant_x_qdd_c1c90/1 -> Subtract_33998/2
  Constant_x_l_3eb2d/1 -> Product_2f50c/2
  Divide_c7b3e/1 -> Blockout_d_psi_kq_SG_D_2_b6d40/1
  State_psi_gq_SG_D_2_8a6ac/1 -> Product_b9aec/1
  Add_b0455/1 -> Product_b9aec/2
  Product_e50dd/1 -> Add_da69a/1
  Constant_x_qd_98b8a/1 -> Add_da69a/2
  Product_dfb4a/1 -> Divide_80bed/1
  State_psi_kq_SG_D_2_dff77/1 -> Product_e73d5/1
  Subtract_33998/1 -> Product_e73d5/2
  Product_2f50c/1 -> Add_95af3/1
  Constant_x_qd_fc460/1 -> Add_95af3/2
  Product_e73d5/1 -> Divide_679ed/1
  Product_b9aec/1 -> Divide_84aa8/1
  Add_da69a/1 -> Divide_84aa8/2
  Add_95af3/1 -> Divide_679ed/2
  State_psi_q_SG_D_2_e662c/1 -> Add_baf6a/2
  Constant_-1_cf773/1 -> Product_35aaa/1
  Constant_x_l_b8f3c/1 -> Product_35aaa/2
  Divide_84aa8/1 -> Subtract_2808a/1
  Divide_679ed/1 -> Subtract_2808a/2
  Product_35aaa/1 -> Add_cf74d/1
  Constant_x_qd_683e6/1 -> Add_cf74d/2
  Subtract_2808a/1 -> Add_baf6a/1
  Constant_x_qdd_6591c/1 -> Divide_80bed/2
  Constant_-1_50411/1 -> Product_0abff/1
  State_psi_gq_SG_D_2_2a2b4/1 -> Product_0abff/2
  Add_cf74d/1 -> Product_dfb4a/1
  Add_baf6a/1 -> Product_dfb4a/2
  Product_0abff/1 -> Subtract_94387/1
  Subtract_94387/1 -> Add_c1458/1
  Divide_80bed/1 -> Add_c1458/2
  Add_c1458/1 -> Divide_c7b3e/1

== system IEEE9Buses/SG_D_2/d_psi_q_SG_D_2_block ==
  note: d_psi_q_SG_D_2 in SG9
      | $2\,\pi \,f_{0}\,\left(v_{d,\mathrm{SG},D,2}\,\cos\left(\theta _{\mathrm{SG},D,2}\right)+v_{q,\mathrm{SG},D,2}\,\sin\left(\theta _{\mathrm{SG},D,2}\right)-\frac{R_{a}\,\left(\psi _{q,\mathrm{SG},D,2}+\frac{\psi _{\mathrm{gq},\mathrm{SG},D,2}\,\left(x_{l}-x_{\mathrm{qdd}}\right)}{x_{l}-x_{\mathrm{qd}}}+\frac{\psi _{\mathrm{kq},\mathrm{SG},D,2}\,\left(x_{\mathrm{qd}}-x_{\mathrm{qdd}}\right)}{x_{l}-x_{\mathrm{qd}}}\right)}{x_{\mathrm{qdd}}}-\frac{\psi _{d,\mathrm{SG},D,2}\,w_{\mathrm{SG},D,2}}{2\,f_{0}\,\pi }\right)$
      | Automatically generated on 2025-09-12 21:32:03 .
  State_psi_gq_SG_D_2_3b9dd : Inport
  State_psi_kq_SG_D_2_534a3 : Inport  Port=2
  State_psi_q_SG_D_2_db54d : Inport  Port=3
  Input_v_d_SG_D_2_f72d1 : Inport  Port=4
  State_theta_SG_D_2_4b6fa : Inport  Port=5
  Input_v_q_SG_D_2_1bb17 : Inport  Port=6
  State_theta_SG_D_2_9667b : Inport  Port=7
  State_psi_d_SG_D_2_ede2a : Inport  Port=8
  State_w_SG_D_2_3e2aa : Inport  Port=9
  Add_97b21 : Sum
  Add_a5023 : Sum
  Add_b4725 : Sum
  Add_d4b98 : Sum
  Add_e3950 : Sum
  Constant_-1_323f0 : Constant  Value=-1
  Constant_-1_4bbe8 : Constant  Value=-1
  Constant_-1_72731 : Constant  Value=-1
  Constant_-2.0_0d2de : Constant  Value=-2.0
  Constant_2.0_1fe7d : Constant  Value=2.0
  Constant_R_a_4ee9a : Constant  Value=R_a
  Constant_f0_14c82 : Constant  Value=f0
  Constant_f0_a7c81 : Constant  Value=f0
  Constant_pi_79d64 : Constant  Value=pi
  Constant_pi_f5e2b : Constant  Value=pi
  Constant_x_l_5a393 : Constant  Value=x_l
  Constant_x_l_6cdca : Constant  Value=x_l
  Constant_x_l_6ec2f : Constant  Value=x_l
  Constant_x_qd_bf3a1 : Constant  Value=x_qd
  Constant_x_qd_f10b2 : Constant  Value=x_qd
  Constant_x_qd_fbd73 : Constant  Value=x_qd
  Constant_x_qdd_25411 : Constant  Value=x_qdd
  Constant_x_qdd_2cf33 : Constant  Value=x_qdd
  Constant_x_qdd_58c11 : Constant  Value=x_qdd
  Divide_4e07d : Product  Inputs=*/
  Divide_909a5 : Product  Inputs=*/
  Divide_b8133 : Product  Inputs=*/
  Divide_e90b1 : Product  Inputs=*/
  MathFunc_cos_e73a6 : Trigonometry  Operator=cos
  MathFunc_sin_7aaf2 : Trigonometry
  Product_0398e : Product
  Product_422f7 : Product
  Product_46b4d : Product
  Product_51916 : Product
  Product_63ac1 : Product
  Product_6f5e0 : Product
  Product_78cd8 : Product
  Product_7bef1 : Product
  Product_7f685 : Product
  Product_a6c56 : Product
  Product_d4203 : Product
  Product_e0abe : Product
  Product_eece5 : Product
  Product_f0f17 : Product
  Subtract_4adf1 : Sum  Inputs=+-
  Subtract_8874d : Sum  Inputs=+-
  Subtract_a6f01 : Sum  Inputs=+-
  Subtract_d5700 : Sum  Inputs=+-
  Blockout_d_psi_q_SG_D_2_456f3 : Outport
  wires:
  Constant_x_qdd_2cf33/1 -> Subtract_4adf1/2
  Constant_x_l_6ec2f/1 -> Product_f0f17/2
  Constant_-1_4bbe8/1 -> Product_e0abe/1
  Constant_x_l_6cdca/1 -> Product_e0abe/2
  Product_e0abe/1 -> Add_b4725/1
  Constant_pi_f5e2b/1 -> Product_eece5/2
  State_psi_gq_SG_D_2_3b9dd/1 -> Product_46b4d/1
  Constant_x_l_5a393/1 -> Product_d4203/2
  State_w_SG_D_2_3e2aa/1 -> Product_7bef1/2
  Constant_x_qd_bf3a1/1 -> Add_a5023/2
  Constant_x_qdd_25411/1 -> Add_b4725/2
  Constant_2.0_1fe7d/1 -> Product_eece5/1
  Constant_-1_72731/1 -> Product_d4203/1
  Constant_x_qd_f10b2/1 -> Subtract_4adf1/1
  Constant_-1_323f0/1 -> Product_f0f17/1
  State_psi_q_SG_D_2_db54d/1 -> Add_97b21/2
  Add_b4725/1 -> Product_46b4d/2
  Product_eece5/1 -> Product_422f7/1
  Product_d4203/1 -> Add_d4b98/1
  Constant_pi_79d64/1 -> Product_6f5e0/2
  Constant_f0_a7c81/1 -> Product_422f7/2
  Constant_x_qd_fbd73/1 -> Add_d4b98/2
  State_psi_kq_SG_D_2_534a3/1 -> Product_63ac1/1
  Subtract_4adf1/1 -> Product_63ac1/2
  Product_f0f17/1 -> Add_a5023/1
  Input_v_q_SG_D_2_1bb17/1 -> Product_51916/1
  Product_46b4d/1 -> Divide_909a5/1
  Product_422f7/1 -> Divide_4e07d/2
  Add_d4b98/1 -> Divide_909a5/2
  Product_63ac1/1 -> Divide_b8133/1
  Add_a5023/1 -> Divide_b8133/2
  Divide_909a5/1 -> Subtract_8874d/1
  State_theta_SG_D_2_4b6fa/1 -> MathFunc_cos_e73a6/1
  Divide_b8133/1 -> Subtract_8874d/2
  Subtract_8874d/1 -> Add_97b21/1
  MathFunc_cos_e73a6/1 -> Product_a6c56/2
  Constant_R_a_4ee9a/1 -> Product_78cd8/1
  Add_97b21/1 -> Product_78cd8/2
  State_theta_SG_D_2_9667b/1 -> MathFunc_sin_7aaf2/1
  Product_78cd8/1 -> Divide_e90b1/1
  Product_6f5e0/1 -> Product_7f685/1
  Product_51916/1 -> Subtract_a6f01/2
  Constant_x_qdd_58c11/1 -> Divide_e90b1/2
  Input_v_d_SG_D_2_f72d1/1 -> Product_a6c56/1
  Add_e3950/1 -> Product_0398e/2
  Divide_e90b1/1 -> Subtract_d5700/1
  Product_a6c56/1 -> Subtract_d5700/2
  MathFunc_sin_7aaf2/1 -> Product_51916/2
  Product_0398e/1 -> Blockout_d_psi_q_SG_D_2_456f3/1
  State_psi_d_SG_D_2_ede2a/1 -> Product_7bef1/1
  Constant_-2.0_0d2de/1 -> Product_6f5e0/1
  Product_7f685/1 -> Product_0398e/1
  Subtract_d5700/1 -> Subtract_a6f01/1
  Product_7bef1/1 -> Divide_4e07d/1
  Constant_f0_14c82/1 -> Product_7f685/2
  Subtract_a6f01/1 -> Add_e3950/1
  Divide_4e07d/1 -> Add_e3950/2

== system IEEE9Buses/SG_D_2/d_theta_SG_D_2_block ==
  note: d_theta_SG_D_2 in SG9
      | $w_{\mathrm{SG},D,2}-2\,\pi \,f_{0}$
      | Automatically generated on 2025-09-12 21:32:27 .
  State_w_SG_D_2_ade08 : Inport
  Add_f39a4 : Sum
  Constant_-2.0_7fab3 : Constant  Value=-2.0
  Constant_f0_4aff8 : Constant  Value=f0
  Constant_pi_687aa : Constant  Value=pi
  Product_355da : Product
  Product_d3dca : Product
  Blockout_d_theta_SG_D_2_0ad08 : Outport
  wires:
  Constant_-2.0_7fab3/1 -> Product_355da/1
  Constant_pi_687aa/1 -> Product_355da/2
  Add_f39a4/1 -> Blockout_d_theta_SG_D_2_0ad08/1
  Product_355da/1 -> Product_d3dca/1
  Constant_f0_4aff8/1 -> Product_d3dca/2
  Product_d3dca/1 -> Add_f39a4/1
  State_w_SG_D_2_ade08/1 -> Add_f39a4/2
